simulink subsystem "Hagglund_Decoupler"  (R2023b)
settings: Solver=VariableStepAuto  StartTime=0.0  StopTime=10.0  RelTol=1e-3
values from neighbouring files (symbols this model uses):
  KF1 = 0    [init_hagglund_models.m]
  KF2 = 0    [init_hagglund_models.m]
settings Model: Creator=HP  LastModifiedBy=HP

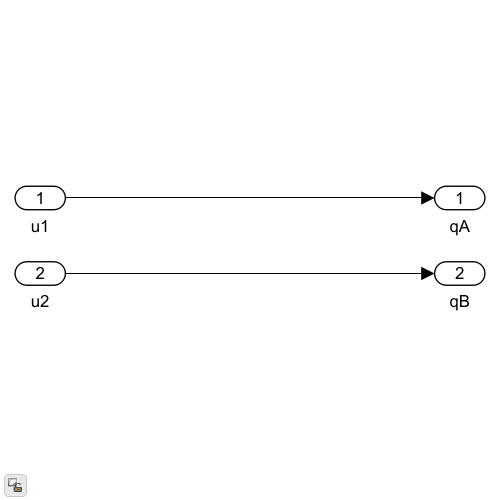
[thumbnail: Simulink's stored preview of the top-level diagram]
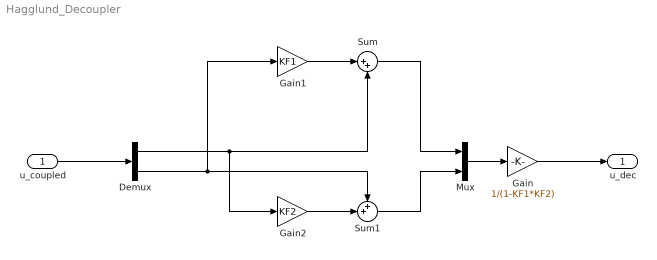
== system Hagglund_Decoupler ==
  u_coupled : Inport
  Demux : Demux  Outputs=2
  Gain : Gain  Gain=1/(1-KF1*KF2)
  Gain1 : Gain  Gain=KF1
  Gain2 : Gain  Gain=KF2
  Mux : Mux  Inputs=2
  Sum : Sum  Inputs=|++
  Sum1 : Sum  Inputs=++|
  u_dec : Outport
  wires:
  Gain/1 -> u_dec/1
  u_coupled/1 -> Demux/1
  Mux/1 -> Gain/1
  Gain1/1 -> Sum/1
  Sum/1 -> Mux/1
  Demux/2 -> Gain1/1, Sum1/1
  Demux/1 -> Sum/2, Gain2/1
  Gain2/1 -> Sum1/2
  Sum1/1 -> Mux/2
